simulink model "lqr_control_alphasat"  (R2023a)
settings: Solver=VariableStepAuto  StartTime=0.0  StopTime=10000  RelTol=1e-3  EnableMultiTasking=on
InitFcn:
  | load('lqr_gain','-mat');
model workspace: external: MAT-File (data not in the file)
libraries: aausat3_lib x13, simulink_extras x2, vrlib x1
settings Model: Creator=jn  LastModifiedBy=jacobel-omar
settings SolverCC: AlgebraicLoopSolver=TrustRegion
settings DataIOCC: SaveFormat=Array  ReturnWorkspaceOutputs=off
settings OptimizationCC: LifeSpan=inf
settings DebuggingCC: SolverPrmCheckMsg=warning  UnconnectedInputMsg=warning  UnconnectedOutputMsg=warning  UnconnectedLineMsg=warning  AllowSymbolicDim=off  SFUnexpectedBacktrackingDiag=warning  SFNoUnconditionalDefaultTransitionDiag=warning  SFExecutionAtInitializationDiag=none  ArithmeticOperatorsInVariantConditions=warning
settings ModelReferenceCC: EnableRefExpFcnMdlSchedulingChecks=on  PropagateSignalLabelsOutOfModel=off
settings SFSimCC: SimUseLocalCustomCode=off  CustomCodeUndefinedFunction=UseInterfaceOnly
settings RTWCC: RTWUseLocalCustomCode=off
settings CodeAppCC: StateflowObjectComments=on
settings GRTTargetCC: TargetLangStandard=C89/C90 (ANSI)
settings ConfigComp: CovMetricSettings=dw  CovSaveCumulativeToWorkspaceVar=on  CovSaveSingleToWorkspaceVar=on  CovExternalEMLEnable=off  CovSFcnEnable=off

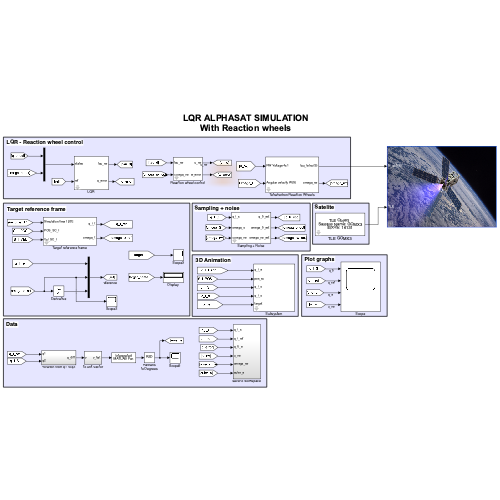
[thumbnail: Simulink's stored preview of the top-level diagram]
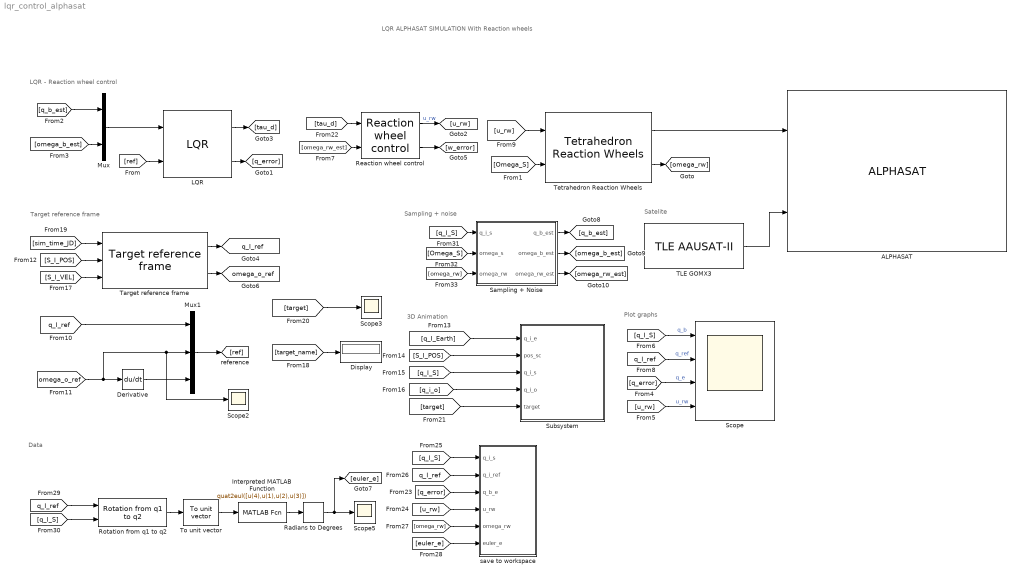
== system lqr_control_alphasat ==
  note: Satelite
  note: Data
  note: Sampling + noise
  note: Target reference frame
  note: Plot graphs
  note: LQR - Reaction wheel control
  note: LQR ALPHASAT SIMULATION
      | With Reaction wheels
  note: 3D Animation
  ALPHASAT : aausat3_lib/ALPHASAT  date='2015-10-20T14:35Z'  q_init_I_S="-[0.5643 -0.1938  0.7691 -0.2289]"  w_init_S=ones(1,3)*deg2rad(0.3)  enable_env_disturbance=on  Dim=[0.1 0.1 0.133]  sc_mass=0.8  r_com=[-5.238e-8, -0.007e-3, -1.394e-3]  inertia_C=[0.6714 0.7044 0.7268]*1e-3  q_S_C=[0.0218,-0.0064, -0.0153, 0.9996]  Cd=2  rho=5e-14  solar_m_flux=4.5565e-6  solar_absorb_coeff=1.5  mag_dipole=0.001
      settings: SourceProductName=AAUSAT3
  Derivative : Derivative
  Display : Display
  Interpreted MATLAB Function : MATLABFcn  MATLABFcn=quat2eul([u(4),u(1),u(2),u(3)])
  LQR : aausat3_lib/ACS/LQR  lqr=K_lqr  q_b_tetra=[0 0 1 0]'  q_s_c=[0.0218,-0.0064, -0.0153, 0.9996]'  Ts=1
      settings: SourceProductName=AAUSAT3
  Mux : Mux  Inputs=2
  Mux1 : Mux  Inputs=3
  Radians to Degrees : simulink_extras/Transformations/Radians to Degrees
  Reaction wheel control : aausat3_lib/ACS/Reaction wheel control  omega_bias=800  Kp=0.0018  Ki=0.004  Ts=1/4  u_bias=3.3/2  Jrw=0.336e-6
      settings: SourceProductName=AAUSAT3
  Rotation from q1 to q2 : aausat3_lib/Math Utilities/Quaternion operations/Rotation from q1 to q2  SystemSampleTime=-1  VariantActivationTime=update diagram  Latency=0  AutoFrameSizeCalculation=off
      settings: SourceProductName=AAUSAT3
  Sampling + Noise : Subsystem  mask{Ts=1}
      mask prompts: Ts "Sampling time [s]"
  Scope : Scope  NumInputPorts=4
  Scope2 : Scope
  Scope3 : Scope
  Scope5 : Scope
  Subsystem : Subsystem  mask{Re=6371e3, scale=1000}
      mask prompts: Re "Earth Radius"; scale "Animation scale"
  TLE GOMX3 : aausat3_lib/Orbit and Ephemeris/TLE AAUSAT-II  satname='GOMX3'  JulianDay=16131.17243197  xndt2o=0.00049328  xndd6o=0  bstar=0.32059e-3  xincl=51.6335  xnodeo=230.6137  eo=0.0003739  omegao=51.3487  xmo=308.7846  xno=15.75443623  ts=1
      settings: SourceProductName=AAUSAT3
  Target reference frame : aausat3_lib/Orbit and Ephemeris/Target reference frame  min_elevation=5  Ts=5  target_list='target_list.mat'  enabel_target=on
      settings: SourceProductName=AAUSAT3
  Tetrahedron Reaction Wheels : aausat3_lib/Actuator Emulation/Tetrahedron Reaction Wheels  q_S_Tetra=[0 0 1 0]  I_w=diag([0.4513 0.4513 0.336])*1e-6  coriolis_on=on  init_omega=800  Kt=1.81e-3  Ke=1.81e-3  Ra=4.44  Vcc=3.3
      settings: SourceProductName=AAUSAT3
  To unit vector : aausat3_lib/Math Utilities/Vector operations/To unit vector  SystemSampleTime=-1  VariantActivationTime=update diagram  Latency=0  AutoFrameSizeCalculation=off
      settings: SourceProductName=AAUSAT3
  save to workspace : Subsystem
  tag scope: omega_o_ref=global, q_I_ref=global
  wires:
  [q_I_ref] -> Mux1/1
  Derivative/1 -> Mux1/3
  [q_I_S] -> Scope/1  "q_b"
  Mux1/1 -> [ref]
  [q_I_ref] -> Scope/2  "q_ref"
  TLE GOMX3/1 -> ALPHASAT/2
  [omega_o_ref] -> Derivative/1, Scope2/1, Mux1/2
  Target reference frame/1 -> [q_I_ref]
  [S_I_VEL] -> Target reference frame/3
  [S_I_POS] -> Target reference frame/2
  Target reference frame/2 -> [omega_o_ref]
  [sim_time_JD] -> Target reference frame/1
  [target_name] -> Display/1
  [target] -> Scope3/1
  [q_I_Earth] -> Subsystem/1(q_i_e)
  [S_I_POS] -> Subsystem/2(pos_sc)
  [q_I_S] -> Subsystem/3(q_i_s)
  [q_i_o] -> Subsystem/4(q_i_o)
  [target] -> Subsystem/5(target)
  [ref] -> LQR/2
  Mux/1 -> LQR/1
  Tetrahedron Reaction Wheels/1 -> ALPHASAT/1
  [q_b_est] -> Mux/1
  [omega_b_est] -> Mux/2
  LQR/2 -> [q_error]
  [q_error] -> Scope/3  "q_e"
  [u_rw] -> Scope/4  "u_rw"
  [Omega_S] -> Tetrahedron Reaction Wheels/2
  Tetrahedron Reaction Wheels/2 -> [omega_rw]
  [omega_rw_est] -> Reaction wheel control/2
  Reaction wheel control/1 -> [u_rw]  "u_rw"
  [u_rw] -> Tetrahedron Reaction Wheels/1
  LQR/1 -> [tau_d]
  [tau_d] -> Reaction wheel control/1
  Reaction wheel control/2 -> [w_error]
  [q_I_ref] -> Rotation from q1 to q2/1
  [q_I_S] -> Rotation from q1 to q2/2
  Rotation from q1 to q2/1 -> To unit vector/1
  To unit vector/1 -> Interpreted MATLAB Function/1
  Interpreted MATLAB Function/1 -> Radians to Degrees/1
  [q_I_S] -> save to workspace/1(q_i_s)
  [q_I_ref] -> save to workspace/2(q_i_ref)
  [q_error] -> save to workspace/3(q_b_e)
  [u_rw] -> save to workspace/4(u_rw)
  [omega_rw] -> save to workspace/5(omega_rw)
  [euler_e] -> save to workspace/6("euler_e ")
  Radians to Degrees/1 -> [euler_e], Scope5/1
  [q_I_S] -> Sampling + Noise/1(q_i_s)
  [Omega_S] -> Sampling + Noise/2(omega_s)
  [omega_rw] -> Sampling + Noise/3(omega_rw)
  Sampling + Noise/1(q_b_est) -> [q_b_est]
  Sampling + Noise/2(omega_b_est) -> [omega_b_est]
  Sampling + Noise/3(omega_rw_est) -> [omega_rw_est]

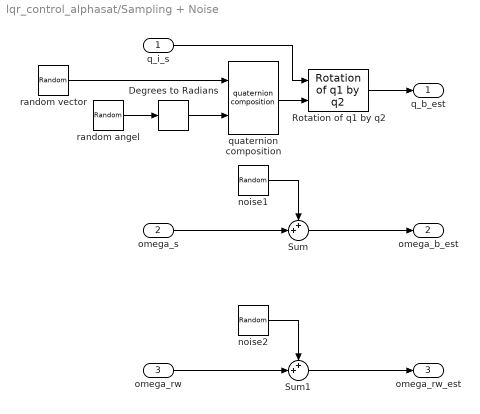
== system lqr_control_alphasat/Sampling + Noise ==
  q_i_s : Inport
  omega_s : Inport  Port=2
  omega_rw : Inport  Port=3
  Degrees to Radians : simulink_extras/Transformations/Degrees to Radians
  Rotation of q1 by q2 : aausat3_lib/Math Utilities/Quaternion operations/Rotation of q1 by q2  SystemSampleTime=-1  VariantActivationTime=update diagram  Latency=0  AutoFrameSizeCalculation=off
      settings: SourceProductName=AAUSAT3
  Sum : Sum  Inputs=++|
  Sum1 : Sum  Inputs=++|
  noise1 : RandomNumber  Mean=zeros(3,1)  Variance=ones(3,1)*0.00012  Seed=[123 1231 54]'
  noise2 : RandomNumber  Mean=zeros(4,1)  Variance=ones(4,1)*0.1  Seed=[34 50 30 23]'
  quaternion composition : aausat3_lib/Math Utilities/Quaternion operations/quaternion composition  SystemSampleTime=-1  VariantActivationTime=update diagram  Latency=0  AutoFrameSizeCalculation=off
      settings: SourceProductName=AAUSAT3
  random angel : RandomNumber  Variance=6.25  Seed=76
  random vector : RandomNumber  Mean=zeros(3,1)  Variance=ones(3,1)  Seed=[45 23 67]'
  q_b_est : Outport
  omega_b_est : Outport  Port=2
  omega_rw_est : Outport  Port=3
  wires:
  random angel/1 -> Degrees to Radians/1
  q_i_s/1 -> Rotation of q1 by q2/1
  Degrees to Radians/1 -> quaternion composition/2
  omega_s/1 -> Sum/2
  noise1/1 -> Sum/1
  omega_rw/1 -> Sum1/2
  noise2/1 -> Sum1/1
  Rotation of q1 by q2/1 -> q_b_est/1
  Sum/1 -> omega_b_est/1
  Sum1/1 -> omega_rw_est/1
  quaternion composition/1 -> Rotation of q1 by q2/2
  random vector/1 -> quaternion composition/1

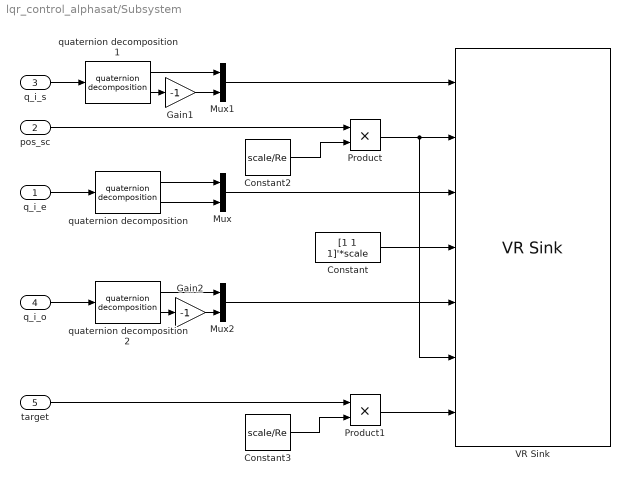
== system lqr_control_alphasat/Subsystem ==
  q_i_e : Inport
  pos_sc : Inport  Port=2
  q_i_s : Inport  Port=3
  q_i_o : Inport  Port=4
  target : Inport  Port=5
  Constant : Constant  Value=[1 1 1]'*scale
  Constant2 : Constant  Value=scale/Re
  Constant3 : Constant  Value=scale/Re
  Gain1 : Gain  Gain=-1
  Gain2 : Gain  Gain=-1
  Mux : Mux  Inputs=2
  Mux1 : Mux  Inputs=2
  Mux2 : Mux  Inputs=2
  Product : Product
  Product1 : Product
  VR Sink : vrlib/VR Sink  InstantiateOnLoad=on  SampleTime=0.1  ViewEnable=on  RemoteChange=off  RemoteView=on  FieldsWritten=CubeSat.rotation.4.1.1.double#CubeSat.translation.3.1.1.double#Earth.rotation.4.1.1.double#trans.scale.3.1.1.double#sat_view.rotation.4.1.1.double#sat_view.translation.3.1.1.double#target.translation.3.1.1.double  WorldFileName=lib/utils/animation/sat_orbit.wrl  WorldDescription=The Earth - Low Resolution Model  AutoView=off  VideoDimensions=[]  AllowVariableSize=off
  quaternion decomposition : aausat3_lib/Math Utilities/Quaternion operations/quaternion decomposition  SystemSampleTime=-1  VariantActivationTime=update diagram  Latency=0  AutoFrameSizeCalculation=off
      settings: SourceProductName=AAUSAT3
  quaternion decomposition1 : aausat3_lib/Math Utilities/Quaternion operations/quaternion decomposition  SystemSampleTime=-1  VariantActivationTime=update diagram  Latency=0  AutoFrameSizeCalculation=off
      settings: SourceProductName=AAUSAT3
  quaternion decomposition2 : aausat3_lib/Math Utilities/Quaternion operations/quaternion decomposition  SystemSampleTime=-1  VariantActivationTime=update diagram  Latency=0  AutoFrameSizeCalculation=off
      settings: SourceProductName=AAUSAT3
  wires:
  q_i_e/1 -> quaternion decomposition/1
  quaternion decomposition/2 -> Mux/2
  quaternion decomposition/1 -> Mux/1
  q_i_s/1 -> quaternion decomposition1/1
  quaternion decomposition1/2 -> Gain1/1
  quaternion decomposition1/1 -> Mux1/1
  q_i_o/1 -> quaternion decomposition2/1
  quaternion decomposition2/1 -> Mux2/1
  Gain1/1 -> Mux1/2
  quaternion decomposition2/2 -> Gain2/1
  Gain2/1 -> Mux2/2
  Mux1/1 -> VR Sink/1
  Constant/1 -> VR Sink/4
  pos_sc/1 -> Product/1
  Product/1 -> VR Sink/6, VR Sink/2
  Constant2/1 -> Product/2
  Product1/1 -> VR Sink/7
  Constant3/1 -> Product1/2
  Mux2/1 -> VR Sink/5
  Mux/1 -> VR Sink/3
  target/1 -> Product1/1

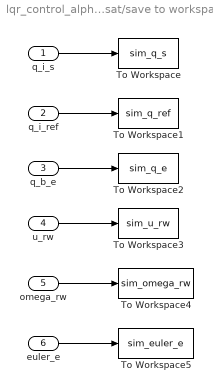
== system lqr_control_alphasat/save to workspace ==
  q_i_s : Inport
  q_i_ref : Inport  Port=2
  q_b_e : Inport  Port=3
  u_rw : Inport  Port=4
  omega_rw : Inport  Port=5
  "euler_e " : Inport  Port=6
  To Workspace : ToWorkspace  VariableName=sim_q_s  SaveFormat=Timeseries  SampleTime=-1
  To Workspace1 : ToWorkspace  VariableName=sim_q_ref  SaveFormat=Timeseries  SampleTime=-1
  To Workspace2 : ToWorkspace  VariableName=sim_q_e  SaveFormat=Timeseries  SampleTime=-1
  To Workspace3 : ToWorkspace  VariableName=sim_u_rw  SaveFormat=Timeseries  SampleTime=-1
  To Workspace4 : ToWorkspace  VariableName=sim_omega_rw  SaveFormat=Timeseries  SampleTime=-1
  To Workspace5 : ToWorkspace  VariableName=sim_euler_e  SaveFormat=Timeseries  SampleTime=-1
  wires:
  q_i_s/1 -> To Workspace/1
  q_i_ref/1 -> To Workspace1/1
  q_b_e/1 -> To Workspace2/1
  u_rw/1 -> To Workspace3/1
  omega_rw/1 -> To Workspace4/1
  "euler_e "/1 -> To Workspace5/1
